simulink model "Problem_1"  (R2020b)
settings: Solver=VariableStepAuto  StartTime=0.0  StopTime=10.0  RelTol=1e-3
values from neighbouring files (symbols this model uses):
  b = 50    [Problem1.m]
  K1 = 50    [Problem1.m]
  K12 = 2000    [Problem1.m]
  M1 = 100    [Problem1.m]
  M2 = 15    [Problem1.m]
settings Model: Creator=Dell  LastModifiedBy=Dell

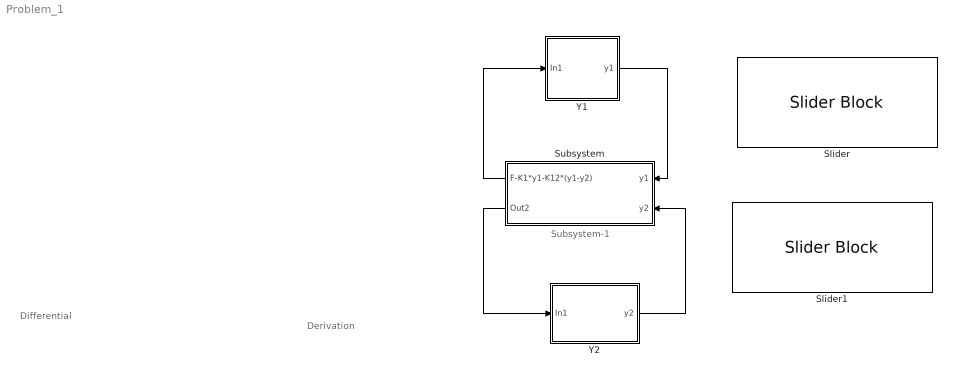
== system Problem_1 ==
  note: Derivation
  note: Differential
  note: Subsystem-1
  Slider : SliderBlock  ScaleMax=2000
  Slider1 : SliderBlock  ScaleMax=50
  Subsystem : Subsystem
  Y1 : Subsystem
  Y2 : Subsystem
  wires:
  Subsystem/1(F-K1*y1-K12*(y1-y2)) -> Y1/1(In1)
  Y1/1(y1) -> Subsystem/1(y1)
  Subsystem/2(Out2) -> Y2/1(In1)
  Y2/1(y2) -> Subsystem/2(y2)

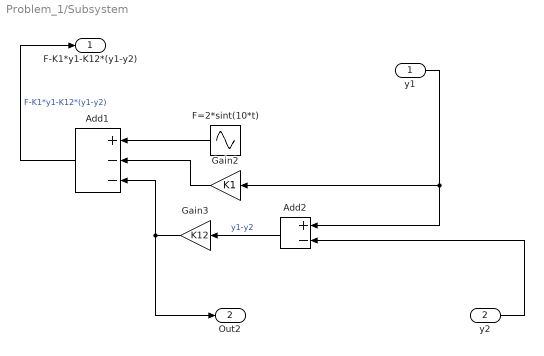
== system Problem_1/Subsystem ==
  y1 : Inport
  y2 : Inport  Port=2
  Add1 : Sum  Inputs=+--
  Add2 : Sum  Inputs=+-
  F=2*sint(10*t) : Sin  Amplitude=2  Frequency=10  SampleTime=0
  Gain2 : Gain  Gain=K1
  Gain3 : Gain  Gain=K12
  F-K1*y1-K12*(y1-y2) : Outport
  Out2 : Outport  Port=2
  wires:
  F=2*sint(10*t)/1 -> Add1/1
  Gain2/1 -> Add1/2
  Gain3/1 -> Out2/1, Add1/3
  y1/1 -> Gain2/1, Add2/1
  y2/1 -> Add2/2
  Add2/1 -> Gain3/1  "y1-y2"
  Add1/1 -> F-K1*y1-K12*(y1-y2)/1  "F-K1*y1-K12*(y1-y2)"

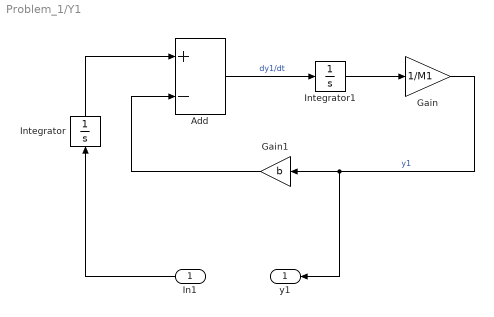
== system Problem_1/Y1 ==
  In1 : Inport
  Add : Sum  Inputs=+-
  Gain : Gain  Gain=1/M1
  Gain1 : Gain  Gain=b
  Integrator : Integrator
  Integrator1 : Integrator
  y1 : Outport
  wires:
  Gain1/1 -> Add/2
  Integrator/1 -> Add/1
  Add/1 -> Integrator1/1  "dy1/dt"
  Gain/1 -> y1/1, Gain1/1  "y1"
  Integrator1/1 -> Gain/1
  In1/1 -> Integrator/1

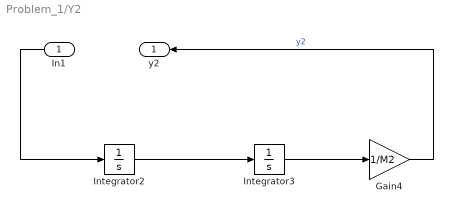
== system Problem_1/Y2 ==
  In1 : Inport
  Gain4 : Gain  Gain=1/M2
  Integrator2 : Integrator
  Integrator3 : Integrator
  y2 : Outport
  wires:
  Integrator3/1 -> Gain4/1
  In1/1 -> Integrator2/1
  Integrator2/1 -> Integrator3/1
  Gain4/1 -> y2/1  "y2"
